simulink model "IP_PID"  (R2015a)
settings: Solver=ode5  StartTime=0.0  StopTime=60  FixedStep=0.01  MaxStep=0.  RelTol=1e-3
libraries: simulink x2
settings Model: Creator=Fares  LastModifiedBy=Fares

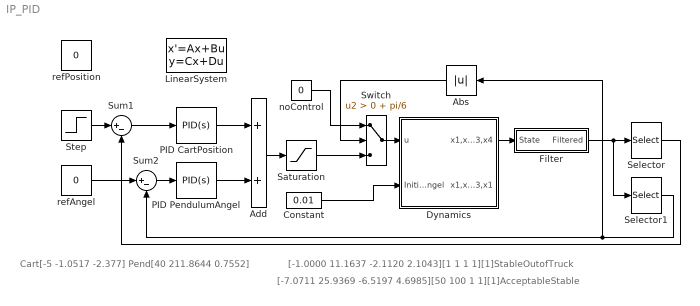
== system IP_PID ==
  note: Cart[-5 -1.0517 -2.377] Pend[40 211.8644 0.7552]
  note: [-7.0711 25.9369 -6.5197 4.6985][50 100 1 1][1]AcceptableStable
  note: [-1.0000 11.1637 -2.1120 2.1043][1 1 1 1][1]StableOutofTruck
  Abs : Abs
  Add : Sum
  Constant : Constant  Value=0.01
  Dynamics : Subsystem  mask{mc=1.12, mpw=0.095, mps=0.025, M=9.4, fp=0.000107443, J=0.013935418, l=0.033245968, g=9.81}
      mask prompts: mc "Cart mass [kg]"; mpw "Pendulum weight mass [kg]"; mps "Pendulum stick mass [kg]"; M "Maximum control [N]"; fp "Pendulum friction [kg*m2/s]"; J "Moment of inertia [kg*m2]"; l "Distance: axis of rotation-mass center [m]"; g "Gravetational acceleration [m/s2]"
      mask init:
      | mp = mpw + mps;
      | a = l^2 + J/(mc + mp);
      | mi = (mc + mp)*l;
      mask Display: plot([0],[-2.5],[5],[4.5],[0 5],[0 0],[0 5],[0.1 0.1],[0 2],[1 1],[2.5 5],[1 1],[2 2.5 2.5 2 2],[1.25 1.25 0.75 0.75 1.25],[2.25 1.5],[1 -2.5]);
  Filter : Subsystem
  LinearSystem : StateSpace  A=A  B=B  C=C  D=D  X0=[0; 0; 0; 0]  mask(SS MASK){}
      mask init:
      | mc = 1.12;
      | mpw = 0.095;
      | mps = 0.025;
      | l = 0.033245968;
      | fc = 2.53165; % FS = 2.53165; FC = 2.28133
      | fp = 0.000107443;
      | J = 0.013935418;
      | g = 9.81;
      | vf = 9.4/2.5; %Voltage to Motor Force ratio
      | mp = mpw + mps;
      | a = l^2 + J/(mc + mp);
      | mu = (mc + mp)*l;
      | 
      | % theta 0 in upward position
      | % theta pi in downward position
      | s = 1; % 1 when upward  -1 when downward
      | 
      | A = [0          0              1               0;
      |      0          0              0               1;
      |      0      (l*mu*g)/J    -(a*fc)/J    -(l*fp)/J;
      |      0      s*(mu*g)/J    -s*(l*fc)/J    -(fp)/J];
      |  
      | B = [         0;
      |               0;
      |        (vf*a)/J;
      |       (s*vf*l)/J];
      |   
      | C = [1 0 0 0;
      |      0 1 0 0;
      |      0 0 1 0;
      |      0 0 0 1];
      |  
      | D = [0;
      |      0;
      |      0;
      |      0];
  PID CartPosition : simulink/Continuous/PID Controller  Controller=PID  TimeDomain=Continuous-time  SampleTime=-1  IntegratorMethod=Forward Euler  FilterMethod=Forward Euler  Form=Parallel  UseFilter=on  ControllerParametersSource=internal  P=-7.0711  I=-1.0517  D=-6.5197  N=100  InitialConditionSource=internal  InitialConditionForIntegrator=0  InitialConditionForFilter=0  ExternalReset=none  LimitOutput=off  UpperSaturationLimit=inf  LowerSaturationLimit=-inf  LinearizeAsGain=on  AntiWindupMode=none  Kb=1  TrackingMode=off  Kt=1  PParamMin=[]  PParamMax=[]  IParamMin=[]  IParamMax=[]  DParamMin=[]  DParamMax=[]  NParamMin=[]  NParamMax=[]  KbParamMin=[]  KbParamMax=[]  KtParamMin=[]  KtParamMax=[]  POutMin=[]  POutMax=[]  IOutMin=[]  IOutMax=[]  DOutMin=[]  DOutMax=[]  NOutMin=[]  NOutMax=[]  KbOutMin=[]  KbOutMax=[]  KtOutMin=[]  KtOutMax=[]  IntegratorOutMin=[]  IntegratorOutMax=[]  FilterOutMin=[]  FilterOutMax=[]  SumOutMin=[]  SumOutMax=[]  SumI1OutMin=[]  SumI1OutMax=[]  SumI2OutMin=[]  SumI2OutMax=[]  SumI3OutMin=[]  SumI3OutMax=[]  SumDOutMin=[]  SumDOutMax=[]  SaturationOutMin=[]  SaturationOutMax=[]  IntegratorContinuousStateAttributes=''  IntegratorStateMustResolveToSignalObject=off  IntegratorRTWStateStorageClass=Auto  FilterContinuousStateAttributes=''  FilterStateMustResolveToSignalObject=off  FilterRTWStateStorageClass=Auto  DifferentiatorICPrevScaledInput=0  DifferentiatorOutMin=[]  DifferentiatorOutMax=[]
  PID PendulumAngel : simulink/Continuous/PID Controller  Controller=PID  TimeDomain=Continuous-time  SampleTime=-1  IntegratorMethod=Forward Euler  FilterMethod=Forward Euler  Form=Parallel  UseFilter=on  ControllerParametersSource=internal  P=25.9369  I=100.8644  D=4.6985  N=100  InitialConditionSource=internal  InitialConditionForIntegrator=0  InitialConditionForFilter=0  ExternalReset=none  LimitOutput=off  UpperSaturationLimit=inf  LowerSaturationLimit=-inf  LinearizeAsGain=on  AntiWindupMode=none  Kb=1  TrackingMode=off  Kt=1  PParamMin=[]  PParamMax=[]  IParamMin=[]  IParamMax=[]  DParamMin=[]  DParamMax=[]  NParamMin=[]  NParamMax=[]  KbParamMin=[]  KbParamMax=[]  KtParamMin=[]  KtParamMax=[]  POutMin=[]  POutMax=[]  IOutMin=[]  IOutMax=[]  DOutMin=[]  DOutMax=[]  NOutMin=[]  NOutMax=[]  KbOutMin=[]  KbOutMax=[]  KtOutMin=[]  KtOutMax=[]  IntegratorOutMin=[]  IntegratorOutMax=[]  FilterOutMin=[]  FilterOutMax=[]  SumOutMin=[]  SumOutMax=[]  SumI1OutMin=[]  SumI1OutMax=[]  SumI2OutMin=[]  SumI2OutMax=[]  SumI3OutMin=[]  SumI3OutMax=[]  SumDOutMin=[]  SumDOutMax=[]  SaturationOutMin=[]  SaturationOutMax=[]  IntegratorContinuousStateAttributes=''  IntegratorStateMustResolveToSignalObject=off  IntegratorRTWStateStorageClass=Auto  FilterContinuousStateAttributes=''  FilterStateMustResolveToSignalObject=off  FilterRTWStateStorageClass=Auto  DifferentiatorICPrevScaledInput=0  DifferentiatorOutMin=[]  DifferentiatorOutMax=[]
  Saturation : Saturate  UpperLimit=2.5  LowerLimit=-2.5
  Selector : Selector  InputPortWidth=4  Indices=[1]
  Selector1 : Selector  InputPortWidth=4  Indices=[2]
  Step : Step  Time=30  Before=-0.2  After=0.2  SampleTime=0
  Sum1 : Sum  Inputs=|+-
  Sum2 : Sum  Inputs=|+-
  Switch : Switch  Criteria=u2 > Threshold  Threshold=0 + pi/6
  noControl : Constant  Value=0
  refAngel : Constant  Value=0
  refPosition : Constant  Value=0
  wires:
  refAngel/1 -> Sum2/1
  Sum2/1 -> PID PendulumAngel/1
  Sum1/1 -> PID CartPosition/1
  Selector/1 -> Sum1/2
  PID PendulumAngel/1 -> Add/2
  Abs/1 -> Switch/2
  noControl/1 -> Switch/1
  Add/1 -> Saturation/1
  Saturation/1 -> Switch/3
  Selector1/1 -> Abs/1, Sum2/2
  PID CartPosition/1 -> Add/1
  Switch/1 -> Dynamics/1(u)
  Constant/1 -> Dynamics/2(Initial_Angel)
  Dynamics/1(x1,x2,x3,x4) -> Filter/1(State)
  Filter/1(Filtered) -> Selector1/1, Selector/1
  Step/1 -> Sum1/1

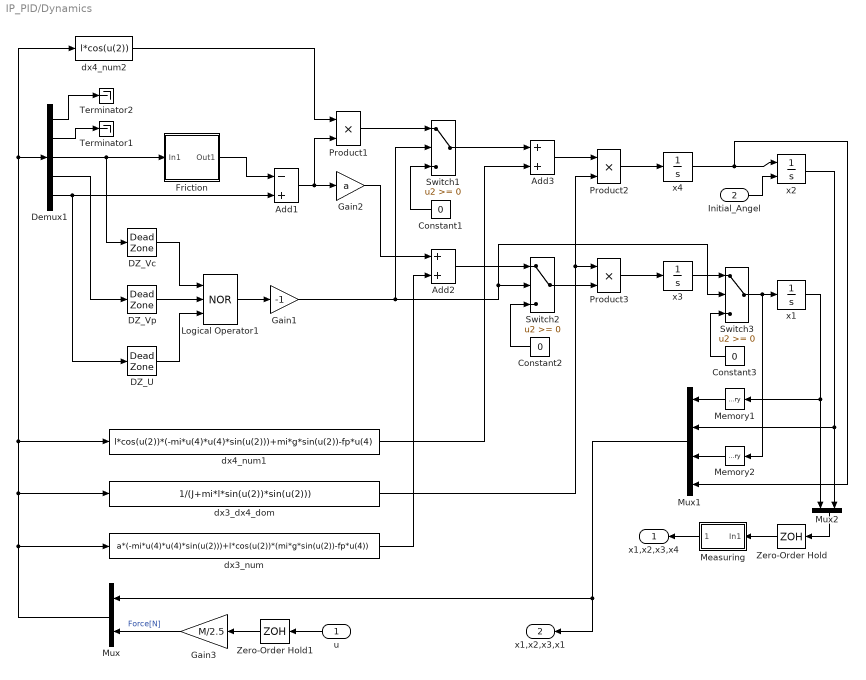
== system IP_PID/Dynamics ==
  u : Inport
  Initial_Angel : Inport  Port=2
  " DZ_Vp" : DeadZone  LowerValue=-3.37476  UpperValue=3.37476  SaturateOnIntegerOverflow=on
  Add1 : Sum  Inputs=-+
  Add2 : Sum
  Add3 : Sum
  Constant1 : Constant  Value=0
  Constant2 : Constant  Value=0
  Constant3 : Constant  Value=0
  DZ_U : DeadZone  LowerValue=-1.37918  UpperValue=1.37918  SaturateOnIntegerOverflow=on
  DZ_Vc : DeadZone  LowerValue=-0.00793711  UpperValue=0.00793711  SaturateOnIntegerOverflow=on
  Demux1 : Demux  Outputs=5
  Friction : Subsystem  mask{FS=2.53165, FC=2.28133, DZcv=0.00793711, Xc=0.9, Yc=2.3}
      mask prompts: FS "Static friction [N]"; FC "Coulombic friction [N]"; DZcv "Minimum cart velocity [rad/s]"; Xc "Cart velocity - beginning of the linear dependence zone [m/s]"; Yc "Friction value for Xc point [N]"
      mask init:
      | small = DZcv;
      mask Display: plot([-4 4],[0 0],[-3.8 -2.4 -1.8 -1.2 -0.6 -0.2 0 0.2 0.6 1.2 1.8 2.4 3.8],[-1.4 -1 -1.1 -1.3 -1.6 -2 0 2 1.6 1.3 1.1 1 1.4]);
  Gain1 : Gain  Gain=-1
  Gain2 : Gain  Gain=a
  Gain3 : Gain  Gain=M/2.5
  Logical Operator1 : Logic  Operator=NOR  Inputs=3  AllPortsSameDT=off  OutDataTypeStr=boolean
  Measuring : Subsystem
  Memory1 : Memory
  Memory2 : Memory
  Mux : Mux  Inputs=2
  Mux1 : Mux
  Mux2 : Mux  Inputs=2
  Product1 : Product
  Product2 : Product
  Product3 : Product
  Switch1 : Switch
  Switch2 : Switch
  Switch3 : Switch
  Terminator1 : Terminator
  Terminator2 : Terminator
  Zero-Order Hold : ZeroOrderHold  SampleTime=0.01
  Zero-Order Hold1 : ZeroOrderHold  SampleTime=0.01
  dx3_dx4_dom : Fcn  Expr=1/(J+mi*l*sin(u(2))*sin(u(2)))
  dx3_num : Fcn  Expr=a*(-mi*u(4)*u(4)*sin(u(2)))+l*cos(u(2))*(mi*g*sin(u(2))-fp*u(4))
  dx4_num1 : Fcn  Expr=l*cos(u(2))*(-mi*u(4)*u(4)*sin(u(2)))+mi*g*sin(u(2))-fp*u(4)
  dx4_num2 : Fcn  Expr=l*cos(u(2))
  x1 : Integrator
  x2 : Integrator  InitialConditionSource=external  InitialCondition=pi/2
  x3 : Integrator
  x4 : Integrator
  x1,x2,x3,x4 : Outport
  x1,x2,x3,x1 : Outport  Port=2
  wires:
  DZ_U/1 -> Logical Operator1/3
  DZ_Vc/1 -> Logical Operator1/1
  Product1/1 -> Switch1/1
  Gain2/1 -> Add2/1
  Constant1/1 -> Switch1/3
  Switch2/1 -> Product3/2
  Product3/1 -> x3/1
  Logical Operator1/1 -> Gain1/1
  Constant3/1 -> Switch3/3
  Add3/1 -> Product2/1
  Demux1/1 -> Terminator2/1
  Mux/1 -> dx3_dx4_dom/1, dx4_num2/1, Demux1/1, dx4_num1/1, dx3_num/1
  dx4_num1/1 -> Add3/2
  x3/1 -> Switch3/1
  Switch3/1 -> Memory2/1, x1/1
  Add1/1 -> Gain2/1, Product1/2
  Add2/1 -> Switch2/1
  dx4_num2/1 -> Product1/1
  Demux1/3 -> Friction/1(In1), DZ_Vc/1
  Demux1/2 -> Terminator1/1
  Demux1/4 -> " DZ_Vp"/1
  Demux1/5 -> Add1/2, DZ_U/1
  " DZ_Vp"/1 -> Logical Operator1/2
  Switch1/1 -> Add3/1
  dx3_num/1 -> Add2/2
  Constant2/1 -> Switch2/3
  dx3_dx4_dom/1 -> Product2/2, Product3/1
  Product2/1 -> x4/1
  x4/1 -> x2/1, Mux1/4
  Memory2/1 -> Mux1/3
  Memory1/1 -> Mux1/1
  Mux1/1 -> x1,x2,x3,x1/1, Mux/1
  u/1 -> Zero-Order Hold1/1
  Friction/1(Out1) -> Add1/1
  Initial_Angel/1 -> x2/2
  Gain1/1 -> Switch1/2, Switch3/2, Switch2/2
  x2/1 -> Mux2/2, Mux1/2
  x1/1 -> Mux2/1, Memory1/1
  Measuring/1(Out1) -> x1,x2,x3,x4/1
  Mux2/1 -> Zero-Order Hold/1
  Zero-Order Hold/1 -> Measuring/1(In1)
  Zero-Order Hold1/1 -> Gain3/1
  Gain3/1 -> Mux/2  "Force[N]"

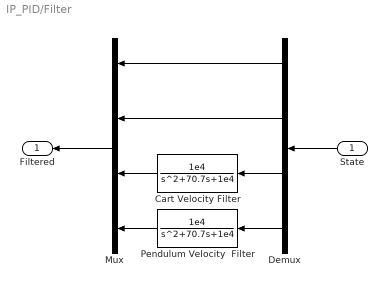
== system IP_PID/Filter ==
  State : Inport
  Cart Velocity Filter : TransferFcn  Numerator=[1e4]  Denominator=[1 70.7 1e4]
  Demux : Demux
  Mux : Mux
  Pendulum Velocity  Filter : TransferFcn  Numerator=[1e4]  Denominator=[1 70.7 1e4]
  Filtered : Outport
  wires:
  Demux/2 -> Mux/2
  State/1 -> Demux/1
  Demux/1 -> Mux/1
  Mux/1 -> Filtered/1
  Cart Velocity Filter/1 -> Mux/3
  Pendulum Velocity  Filter/1 -> Mux/4
  Demux/3 -> Cart Velocity Filter/1
  Demux/4 -> Pendulum Velocity  Filter/1

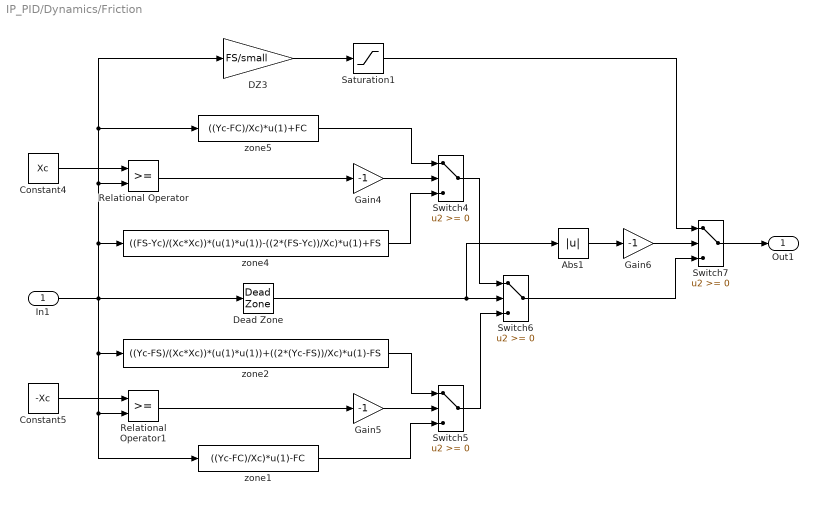
== system IP_PID/Dynamics/Friction ==
  In1 : Inport
  Abs1 : Abs
  Constant4 : Constant  Value=Xc
  Constant5 : Constant  Value=-Xc
  DZ3 : Gain  Gain=FS/small
  Dead Zone : DeadZone  LowerValue=-DZcv  UpperValue=DZcv  SaturateOnIntegerOverflow=on
  Gain4 : Gain  Gain=-1
  Gain5 : Gain  Gain=-1
  Gain6 : Gain  Gain=-1
  Relational Operator : RelationalOperator  OutDataTypeStr=boolean
  Relational Operator1 : RelationalOperator  OutDataTypeStr=boolean
  Saturation1 : Saturate  UpperLimit=FS  LowerLimit=-FS
  Switch{4..7} (4 alike) : Switch
  zone1 : Fcn  Expr=((Yc-FC)/Xc)*u(1)-FC
  zone2 : Fcn  Expr=((Yc-FS)/(Xc*Xc))*(u(1)*u(1))+((2*(Yc-FS))/Xc)*u(1)-FS
  zone4 : Fcn  Expr=((FS-Yc)/(Xc*Xc))*(u(1)*u(1))-((2*(FS-Yc))/Xc)*u(1)+FS
  zone5 : Fcn  Expr=((Yc-FC)/Xc)*u(1)+FC
  Out1 : Outport
  wires:
  Gain4/1 -> Switch4/2
  Dead Zone/1 -> Abs1/1, Switch6/2
  Gain5/1 -> Switch5/2
  Relational Operator/1 -> Gain4/1
  Constant5/1 -> Relational Operator1/1
  Relational Operator1/1 -> Gain5/1
  Abs1/1 -> Gain6/1
  DZ3/1 -> Saturation1/1
  Switch6/1 -> Switch7/3
  Switch4/1 -> Switch6/1
  zone2/1 -> Switch5/1
  Gain6/1 -> Switch7/2
  zone4/1 -> Switch4/3
  Switch7/1 -> Out1/1
  In1/1 -> zone1/1, Relational Operator1/2, zone2/1, DZ3/1, zone5/1, Relational Operator/2, zone4/1, Dead Zone/1
  Saturation1/1 -> Switch7/1
  zone5/1 -> Switch4/1
  Constant4/1 -> Relational Operator/1
  zone1/1 -> Switch5/3
  Switch5/1 -> Switch6/3

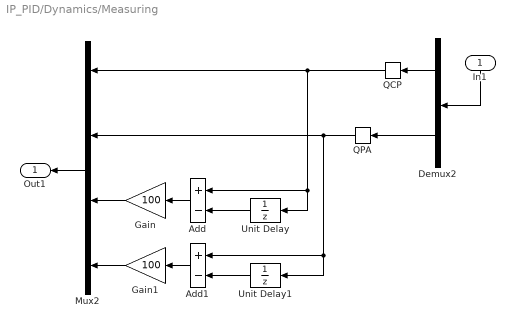
== system IP_PID/Dynamics/Measuring ==
  In1 : Inport
  Add : Sum  Inputs=+-
  Add1 : Sum  Inputs=+-
  Demux2 : Demux  Outputs=2
  Gain : Gain  Gain=100
  Gain1 : Gain  Gain=100
  Mux2 : Mux
  QCP : Quantizer  QuantizationInterval=0.156/2048
  QPA : Quantizer  QuantizationInterval=(2*pi)/2048
  Unit Delay : UnitDelay  SampleTime=-1
  Unit Delay1 : UnitDelay  SampleTime=-1
  Out1 : Outport
  wires:
  Demux2/1 -> QCP/1
  Mux2/1 -> Out1/1
  In1/1 -> Demux2/1
  QPA/1 -> Unit Delay1/1, Add1/1, Mux2/2
  QCP/1 -> Unit Delay/1, Add/1, Mux2/1
  Demux2/2 -> QPA/1
  Unit Delay1/1 -> Add1/2
  Unit Delay/1 -> Add/2
  Add1/1 -> Gain1/1
  Add/1 -> Gain/1
  Gain1/1 -> Mux2/4
  Gain/1 -> Mux2/3
